simulink model "recup"  (R2016b)
settings: Solver=VariableStepAuto  StartTime=0.0  StopTime=10.0  RelTol=1e-3
settings Model: Creator=Julian Ulrich  LastModifiedBy=Julian Ulrich

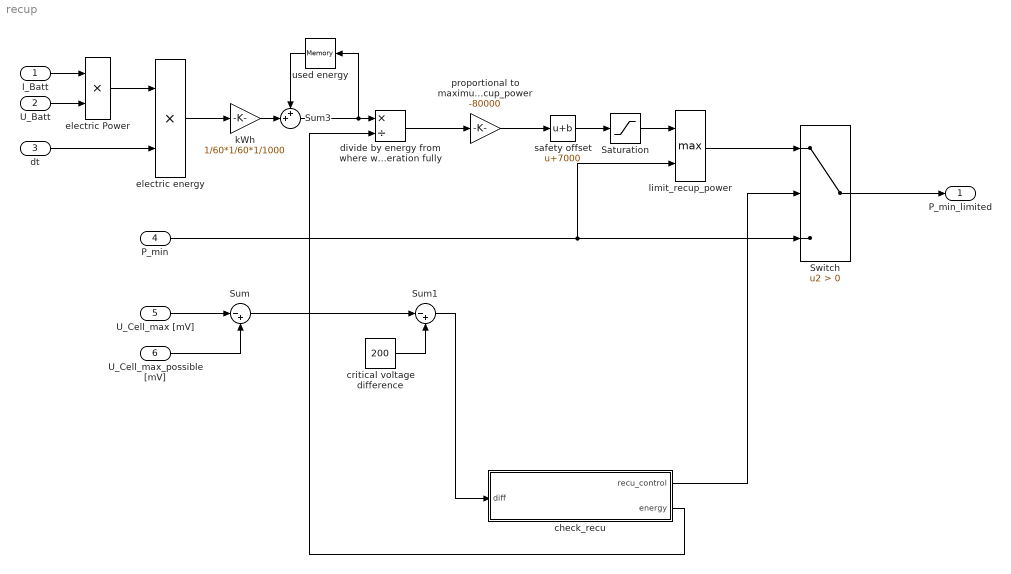
== system recup ==
  I_Batt : Inport
  U_Batt : Inport  Port=2
  dt : Inport  Port=3
  P_min : Inport  Port=4
  U_Cell_max [mV] : Inport  Port=5
  U_Cell_max_possible [mV] : Inport  Port=6
  Saturation : Saturate  UpperLimit=0  LowerLimit=-100000
  Sum : Sum  Inputs=|-+
  Sum1 : Sum  Inputs=|-+
  Sum3 : Sum  Inputs=++|
  Switch : Switch  Criteria=u2 > Threshold
  check_recu : MATLAB Function  TreatAsAtomicUnit=on
  "critical voltage difference " : Constant  Value=200
  divide by energy from where we can use recuperation fully : Product  Inputs=*/
  electric Power : Product
  electric energy : Product
  kWh : Gain  Gain=1/60*1/60*1/1000
  limit_recup_power : MinMax  Function=max  Inputs=2
  proportional to maximum_recup_power : Gain  Gain=-80000
  safety offset : Bias  Bias=7000
  used energy : Memory  InheritSampleTime=on
  P_min_limited : Outport
  wires:
  U_Cell_max_possible [mV]/1 -> Sum/2
  Sum/1 -> Sum1/1
  "critical voltage difference "/1 -> Sum1/2
  P_min/1 -> limit_recup_power/2, Switch/3
  I_Batt/1 -> electric Power/1
  U_Batt/1 -> electric Power/2
  dt/1 -> electric energy/2
  electric Power/1 -> electric energy/1
  electric energy/1 -> kWh/1
  Sum1/1 -> check_recu/1(diff)
  kWh/1 -> Sum3/2
  proportional to maximum_recup_power/1 -> safety offset/1
  check_recu/1(recu_control) -> Switch/2
  Sum3/1 -> divide by energy from where we can use recuperation fully/1, used energy/1
  used energy/1 -> Sum3/1
  Saturation/1 -> limit_recup_power/1
  limit_recup_power/1 -> Switch/1
  safety offset/1 -> Saturation/1
  divide by energy from where we can use recuperation fully/1 -> proportional to maximum_recup_power/1
  check_recu/2(energy) -> divide by energy from where we can use recuperation fully/2
  U_Cell_max [mV]/1 -> Sum/1
  Switch/1 -> P_min_limited/1

== matlab function recup/check_recu ==
  data: diff input; recu_control output; energy output
function [recu_control, energy] = check_recu(diff)

persistent isActive

if isempty(isActive) %evaluated first time
    if diff > 0
        recu_control = 1;
        energy = diff * 0.0036 + eps;
    else
        recu_control = 0;
        energy = eps;
    end
    
    isActive.recu_contr = recu_control;
    isActive.energiemenge  = energy;

else
    recu_control = isActive.recu_contr;
    energy  = isActive.energy;
end
